simulink model "Rocket"  (R2020b)
settings: Solver=ode15s  StartTime=0.0  StopTime=350  RelTol=1e-3
undefined symbols (not defined in the file or in its folder): g, gam_0, gam_in, h_0, m_dot, m_zfw, R_E, t_turn, v_0, x_0
libraries: simulink x1, pid_lib x1
settings Model: Creator=naimishbalaji  LastModifiedBy=naimishbalaji

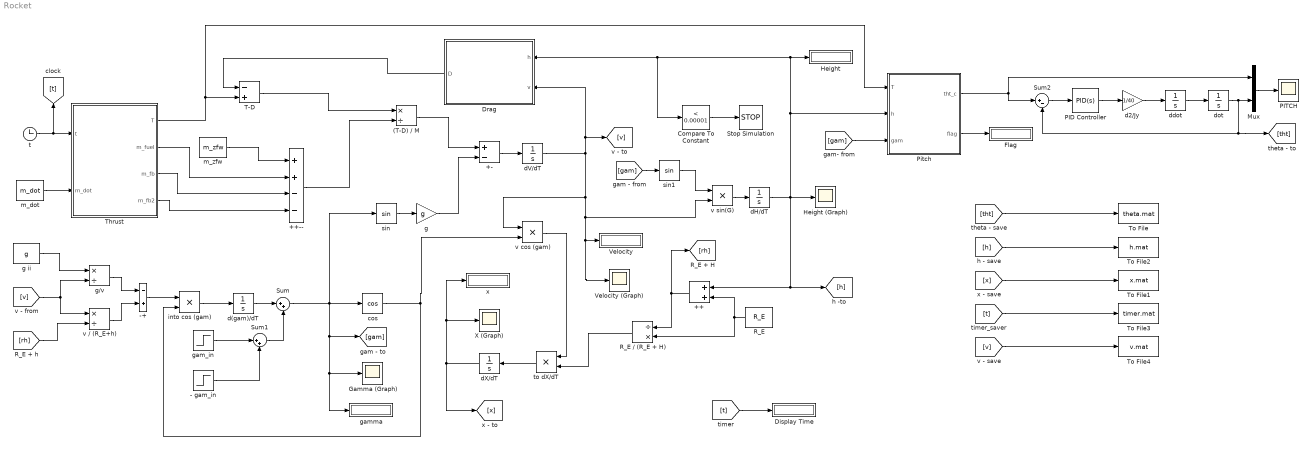
== system Rocket ==
  (T-D) / M : Product  Inputs=*/
  ++ : Sum
  ++-- : Sum  Inputs=++--
  +- : Sum  Inputs=+-
  - gam_in : Step  Time=t_turn + 1  Before=-gam_in  After=-gam_in  SampleTime=0
  -+ : Sum  Inputs=-+
  Compare To Constant : simulink/Logic and Bit Operations/Compare To Constant  relop=<  const=0.00001  OutDataTypeStr=boolean
  Display Time : Display
  Drag : MATLAB Function  TreatAsAtomicUnit=on
  Flag : Display
  Gamma (Graph) : Scope
  Height : Display
  Height (Graph) : Scope
  Mux : Mux  Inputs=2
  PID Controller : pid_lib/PID Controller  Controller=PID  Form=Parallel  TimeDomain=Continuous-time  UseExternalTs=off  SampleTime=-1  IntegratorMethod=Forward Euler  FilterMethod=Forward Euler  ControllerParametersSource=internal  P=0  I=0  D=40  UseFilter=on  N=100  TunerSelectOption=Transfer Function Based (PID Tuner App)  InitialConditionSource=internal  InitialConditionForIntegrator=0  InitialConditionForFilter=0  DifferentiatorICPrevScaledInput=0  ExternalReset=none  TrackingMode=off  Kt=1  LimitOutput=off  SatLimitsSource=internal  UpperSaturationLimit=inf  LowerSaturationLimit=-inf  LinearizeAsGain=on  AntiWindupMode=none  Kb=1  POutMin=[]  POutMax=[]  IOutMin=[]  IOutMax=[]  DOutMin=[]  DOutMax=[]  NOutMin=[]  NOutMax=[]  SumOutMin=[]  SumOutMax=[]  SaturationOutMin=[]  SaturationOutMax=[]  PParamMin=[]  PParamMax=[]  IParamMin=[]  IParamMax=[]  DParamMin=[]  DParamMax=[]  NParamMin=[]  NParamMax=[]  KbParamMin=[]  KbParamMax=[]  KtParamMin=[]  KtParamMax=[]  KbOutMin=[]  KbOutMax=[]  KtOutMin=[]  KtOutMax=[]  IntegratorOutMin=[]  IntegratorOutMax=[]  FilterOutMin=[]  FilterOutMax=[]  SumI1OutMin=[]  SumI1OutMax=[]  SumI2OutMin=[]  SumI2OutMax=[]  SumI3OutMin=[]  SumI3OutMax=[]  SumI4OutMin=[]  SumI4OutMax=[]  SumDOutMin=[]  SumDOutMax=[]  DifferentiatorOutMin=[]  DifferentiatorOutMax=[]  FilterDiffOutCoefMin=[]  FilterDiffOutCoefMax=[]  ReciprocalOutMin=[]  ReciprocalOutMax=[]  SumDenOutMin=[]  SumDenOutMax=[]  SumNumOutMin=[]  SumNumOutMax=[]  DivideOutMin=[]  DivideOutMax=[]  UdiffTsProdOutMin=[]  UdiffTsProdOutMax=[]  NTsProdOutMin=[]  NTsProdOutMax=[]  UintegralTsProdOutMin=[]  UintegralTsProdOutMax=[]  UngainTsProdOutMin=[]  UngainTsProdOutMax=[]  IntegratorContinuousStateAttributes=''  IntegratorStateMustResolveToSignalObject=off  IntegratorRTWStateStorageClass=Auto  FilterContinuousStateAttributes=''  FilterStateMustResolveToSignalObject=off  FilterRTWStateStorageClass=Auto  ParallelPVariant=InternalParameters  IdealPVariant=Disabled  IVariant=InternalParameters  DVariant=InternalParameters  IntegratorVariant=Continuous  SatVariant=Disabled  AWVariant=Passthrough  PCopyVariant=Disabled  TRVariant=Disabled  FdbkBlocksVariant=Forward  IdealPFdbkVariant=Disabled  SatFdbkVariant=Disabled  DerivativeFilterVariant=ContFilter  NVariant=InternalParameters  NCopyVariant=Disabled  FilterICVariant=InternalICsFilter  IntegratorICVariant=InternalICs  ExternalResetVariant=Disabled  TRSumVariant=Passthrough  SumFdbkVariant=Disabled  SumVariant=Sum_PID  TsampFilterVariant=InternalTs  TsampNgainVariant=Passthrough  TsampIntegralVariant=Passthrough  ExternalSaturationOutDataTypeStr=Inherit: Same as second input
  PITCH : Scope
  Pitch : MATLAB Function  TreatAsAtomicUnit=on
  R_E : Constant  Value=R_E
  R_E / (R_E + H) : Product  Inputs=/*
  Stop Simulation : Stop
  Sum : Sum  Inputs=|++
  Sum1 : Sum  Inputs=|++
  Sum2 : Sum  Inputs=|+-
  T-D : Sum  Inputs=-+
  Thrust : MATLAB Function  TreatAsAtomicUnit=on
  To File : ToFile  Filename=theta.mat  MatrixName=tht
  To File1 : ToFile  Filename=x.mat  MatrixName=x
  To File2 : ToFile  Filename=h.mat  MatrixName=h
  To File3 : ToFile  Filename=timer.mat  MatrixName=t
  To File4 : ToFile  Filename=v.mat  MatrixName=v
  Velocity : Display
  Velocity (Graph) : Scope
  X (Graph) : Scope
  cos : Trigonometry  Operator=cos
  d(gam)/dT : Integrator  InitialCondition=gam_0
  d2/Jy : Gain  Gain=1/40
  dH/dT : Integrator  InitialCondition=h_0
  dV/dT : Integrator  InitialCondition=v_0
  dX/dT : Integrator  InitialCondition=x_0
  ddot : Integrator
  dot : Integrator  InitialCondition=pi/2
  g : Gain  Gain=g
  g ii : Constant  Value=g
  g/v : Product  Inputs=*/
  gam_in : Step  Time=t_turn  Before=gam_in  After=0  SampleTime=0
  gamma : Display
  into cos (gam) : Product
  m_dot : Constant  Value=m_dot
  m_zfw : Constant  Value=m_zfw
  sin : Trigonometry
  sin1 : Trigonometry
  t : Clock
  to dX/dT : Product
  v / (R_E+h) : Product  Inputs=*/
  v cos (gam) : Product
  v sin(G) : Product
  x : Display
  wires:
  t/1 -> Thrust/1(t), [t]
  m_dot/1 -> Thrust/2(m_dot)
  Thrust/2(m_fuel) -> ++--/2
  Thrust/3(m_fb) -> ++--/3
  Thrust/4(m_fb2) -> ++--/4
  m_zfw/1 -> ++--/1
  T-D/1 -> (T-D) / M/1
  ++--/1 -> (T-D) / M/2
  (T-D) / M/1 -> +-/1
  g/1 -> +-/2
  sin/1 -> g/1
  +-/1 -> dV/dT/1
  dV/dT/1 -> Velocity (Graph)/1, Velocity/1, v sin(G)/2, v cos (gam)/1, Drag/2(v), [v]
  v sin(G)/1 -> dH/dT/1
  Thrust/1(T) -> Pitch/1(T), T-D/2
  Drag/1(D) -> T-D/1
  Compare To Constant/1 -> Stop Simulation/1
  R_E/1 -> ++/2, R_E / (R_E + H)/2
  ++/1 -> R_E / (R_E + H)/1, [rh]
  R_E / (R_E + H)/1 -> to dX/dT/2
  to dX/dT/1 -> dX/dT/1
  g ii/1 -> g/v/1
  [v] -> g/v/2, v / (R_E+h)/1
  [rh] -> v / (R_E+h)/2
  v / (R_E+h)/1 -> -+/2
  g/v/1 -> -+/1
  into cos (gam)/1 -> d(gam)/dT/1
  d(gam)/dT/1 -> Sum/1
  -+/1 -> into cos (gam)/1
  cos/1 -> v cos (gam)/2, into cos (gam)/2
  v cos (gam)/1 -> to dX/dT/1
  Sum/1 -> cos/1, gamma/1, Gamma (Graph)/1, [gam], sin/1
  [gam] -> sin1/1
  sin1/1 -> v sin(G)/1
  gam_in/1 -> Sum1/1
  - gam_in/1 -> Sum1/2
  Sum1/1 -> Sum/2
  [gam] -> Pitch/3(gam)
  Pitch/2(flag) -> Flag/1
  Pitch/1(tht_c) -> Sum2/1, Mux/1
  Sum2/1 -> PID Controller/1
  PID Controller/1 -> d2/Jy/1
  ddot/1 -> dot/1
  d2/Jy/1 -> ddot/1
  dot/1 -> Mux/2, [tht], Sum2/2
  Mux/1 -> PITCH/1
  [t] -> Display Time/1
  dH/dT/1 -> Drag/1(h), Compare To Constant/1, Height/1, Pitch/2(h), Height (Graph)/1, [h], ++/1
  [tht] -> To File/1
  [h] -> To File2/1
  [x] -> To File1/1
  dX/dT/1 -> x/1, X (Graph)/1, [x]
  [t] -> To File3/1
  [v] -> To File4/1

== matlab function Rocket/Pitch ==
  settings: updateMethod=DISCRETE
  data: T input; h input; tht_c output; gam input; flag output
function [tht_c, flag] = fcn(T, h, gam)

persistent f

if isempty(f)
    f = 0;
end

if T<=0
    t_c = gam+pi;
    if t_c > pi
        t_c = pi;
    end
    f = 1;

elseif (T<=0) && (h<1000)
    t_c = pi/2;

else
    t_c =  gam;
end

flag = f;
tht_c = t_c;

== matlab function Rocket/Thrust ==
  settings: updateMethod=DISCRETE
  data: t input; T output; m_fuel output; m_fb output; m_fb2 output; m_dot input
function [T, m_fuel, m_fb, m_fb2] = fcn(t, m_dot)

persistent mfb
persistent mfb2

if isempty(mfb)
    mfb = 0;
end
if isempty(mfb2)
    mfb2 = 0;
end

mfuel = 21491.26;

if (mfb <= 0.67 * mfuel)
    THR =  346961.2;
    mfb = t * m_dot;
else
    THR = 0;
end

if (125 < t) && (t < 295)
    THR = -110000;
    mfb2 = (t-125)*(m_dot/3);
end

T = THR;
m_fb = mfb;
m_fb2 = mfb2;
m_fuel = mfuel;

== matlab function Rocket/Drag ==
  data: h input; D output; v input
 function D = fcn(h, v)
% Using Standard Atmosphere Model

CD = 0.075;
Di = 1.5;
A = pi*(Di^2)/4;

if h <= 11000
    T = 15.04 - 0.00649*h;
    p = 101.29 * ((T+273.1)/288.8)^5.258;
elseif (11000 < h) && (h <= 25000)
    T = -56.46;
    p = 22.65*exp(1.73-0.008157*h);
else
    T = -131.21 + 0.00299*h;
    p = 2.488 * ((T+273.1)/216.6)^-11.388;
end

rho = p/(0.2869*(T+273.1))
Drag = 0.5 * rho * v * v * A * CD;

D = Drag;
